simulink model "ramadan_2022"  (R2021a)
settings: Solver=ode15s  StartTime=0.0  StopTime=10  MaxStep=1e-2  MinStep=1e-20  RelTol=1e-3
StartFcn:
  | tic
StopFcn:
  | toc
  | 
  | 
  | %if GimbalLockFlag
  |  % fprintf(2, 'Almost reached Gimbal Lock of IMU. Simulation stopped.\n')
  | %end
  | 
  | %fprintf('Elapsed time: %4.2f sec (%4.2f%% realtime)\n', a, tout(end)/a*100)
values from neighbouring files (symbols this model uses):
  Balance = pMod(26:29)    [AssignSimulinkParams.m]    (also in assign_parameters.m = param(26:29))
  BalanceTrunkLat = pMod(22:25)    [AssignSimulinkParams.m]    (also in assign_parameters.m = param(22:25))
  BasisStim = pMod(1:11)    [AssignSimulinkParams.m]    (also in assign_parameters.m = param(1:11))
  CompliantLeg = pMod(12:14)    [AssignSimulinkParams.m]    (also in assign_parameters.m = param(12:14))
  CompliantLegLat = pMod(15)    [AssignSimulinkParams.m]    (also in assign_parameters.m = param(15))
  lp1 = 0.45    [nms3D_prep.m]
  lp2 = 0.55    [nms3D_prep.m]
  N = size(x,1)    [cmaes_hg.m]
  PreventKneeOverextension = pMod(16:21)    [AssignSimulinkParams.m]    (also in assign_parameters.m = param(16:21))
  propulsion = pMod(35)    [AssignSimulinkParams.m]    (also in assign_parameters.m = param(35))
  s = x(1:N-1,:).^2 + x(2:N,:).^2    [cmaes_hg.m]
  Target02 = pMod(30)    [AssignSimulinkParams.m]    (also in assign_parameters.m = param(30))
  Target13 = pMod(31:33)    [AssignSimulinkParams.m]    (also in assign_parameters.m = param(31:33))
  theta0 = pMod(34)    [AssignSimulinkParams.m]    (also in assign_parameters.m = param(34))
  WramameiSL_1000 = readmatrix('WSL_1000_Norm_Sigmoid_MSE_cont.csv')    [nms3D_prep.m]
  ZramameiSL_1000 = readmatrix('ZSL_1000_Norm_Sigmoid_MSE_cont.csv')    [nms3D_prep.m]
undefined symbols (not defined in the file or in its folder): ICs, mParams, X, Y, Z
libraries: nesl_utility x110, sm_lib x88, simulink x79, eeGeneralControl x28, robotmaniplib x10, dspinverses x10, robotcorelib x5, dspmathops x3, pid_lib x2, vrlib x1
(part 6 of 9)

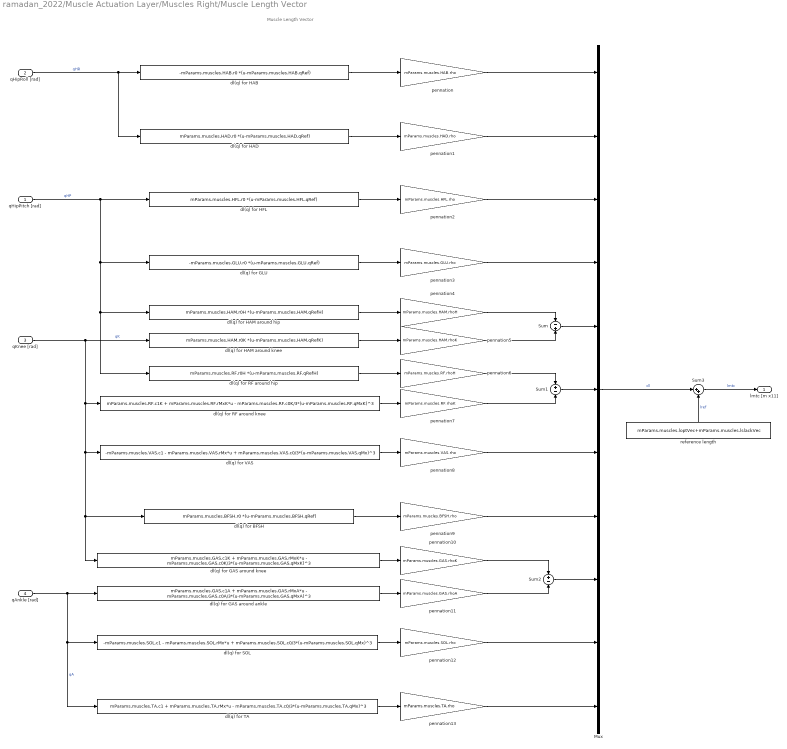
== system ramadan_2022/Muscle Actuation Layer/Muscles Right/Muscle Length Vector ==
  note: Muscle Length Vector
  qHipPitch [rad] : Inport
  qHipRoll [rad] : Inport  Port=2
  qKnee [rad] : Inport  Port=3
  qAnkle [rad] : Inport  Port=4
  Mux : Mux  Inputs=11
  Sum : Sum  Inputs=-+
  Sum1 : Sum  Inputs=+-
  Sum2 : Sum  Inputs=+-
  Sum3 : Sum  Inputs=|++
  dl(q) for BFSH : Fcn  Expr=mParams.muscles.BFSH.r0 *(u-mParams.muscles.BFSH.qRef)
  dl(q) for GAS around ankle : Fcn  Expr=mParams.muscles.GAS.c1A + mParams.muscles.GAS.rMxA*u - mParams.muscles.GAS.c0A/3*(u-mParams.muscles.GAS.qMxA)^3
  dl(q) for GAS around knee : Fcn  Expr=mParams.muscles.GAS.c1K + mParams.muscles.GAS.rMxK*u - mParams.muscles.GAS.c0K/3*(u-mParams.muscles.GAS.qMxK)^3
  dl(q) for GLU : Fcn  Expr=-mParams.muscles.GLU.r0 *(u-mParams.muscles.GLU.qRef)
  dl(q) for HAB : Fcn  Expr=-mParams.muscles.HAB.r0 *(u-mParams.muscles.HAB.qRef)
  dl(q) for HAD : Fcn  Expr=mParams.muscles.HAD.r0 *(u-mParams.muscles.HAD.qRef)
  dl(q) for HAM around hip : Fcn  Expr=mParams.muscles.HAM.r0H *(u-mParams.muscles.HAM.qRefH)
  dl(q) for HAM around knee : Fcn  Expr=mParams.muscles.HAM.r0K *(u-mParams.muscles.HAM.qRefK)
  dl(q) for HFL : Fcn  Expr=mParams.muscles.HFL.r0 *(u-mParams.muscles.HFL.qRef)
  dl(q) for RF around hip : Fcn  Expr=mParams.muscles.RF.r0H *(u-mParams.muscles.RF.qRefH)
  dl(q) for RF around knee : Fcn  Expr=mParams.muscles.RF.c1K + mParams.muscles.RF.rMxK*u - mParams.muscles.RF.c0K/3*(u-mParams.muscles.RF.qMxK)^3
  dl(q) for SOL : Fcn  Expr=-mParams.muscles.SOL.c1 - mParams.muscles.SOL.rMx*u + mParams.muscles.SOL.c0/3*(u-mParams.muscles.SOL.qMx)^3
  dl(q) for TA : Fcn  Expr=mParams.muscles.TA.c1 + mParams.muscles.TA.rMx*u - mParams.muscles.TA.c0/3*(u-mParams.muscles.TA.qMx)^3
  dl(q) for VAS : Fcn  Expr=-mParams.muscles.VAS.c1 - mParams.muscles.VAS.rMx*u + mParams.muscles.VAS.c0/3*(u-mParams.muscles.VAS.qMx)^3
  pennation : Gain  Gain=mParams.muscles.HAB.rho
  pennation1 : Gain  Gain=mParams.muscles.HAD.rho
  pennation10 : Gain  Gain=mParams.muscles.GAS.rhoK
  pennation11 : Gain  Gain=mParams.muscles.GAS.rhoA
  pennation12 : Gain  Gain=mParams.muscles.SOL.rho
  pennation13 : Gain  Gain=mParams.muscles.TA.rho
  pennation2 : Gain  Gain=mParams.muscles.HFL.rho
  pennation3 : Gain  Gain=mParams.muscles.GLU.rho
  pennation4 : Gain  Gain=mParams.muscles.HAM.rhoH
  pennation5 : Gain  Gain=mParams.muscles.HAM.rhoK
  pennation6 : Gain  Gain=mParams.muscles.RF.rhoH
  pennation7 : Gain  Gain=mParams.muscles.RF.rhoK
  pennation8 : Gain  Gain=mParams.muscles.VAS.rho
  pennation9 : Gain  Gain=mParams.muscles.BFSH.rho
  reference length : Constant  Value=mParams.muscles.loptVec+mParams.muscles.lslackVec
  lmtc [m x11] : Outport  VectorParamsAs1DForOutWhenUnconnected=off
  wires:
  dl(q) for HAB/1 -> pennation/1
  dl(q) for HFL/1 -> pennation2/1
  dl(q) for HAM around knee/1 -> pennation5/1
  dl(q) for BFSH/1 -> pennation9/1
  dl(q) for HAM around hip/1 -> pennation4/1
  qAnkle [rad]/1 -> dl(q) for TA/1, dl(q) for SOL/1, dl(q) for GAS around ankle/1  "qA"
  dl(q) for TA/1 -> pennation13/1
  dl(q) for HAD/1 -> pennation1/1
  dl(q) for GLU/1 -> pennation3/1
  dl(q) for RF around knee/1 -> pennation7/1
  dl(q) for SOL/1 -> pennation12/1
  qHipPitch [rad]/1 -> dl(q) for HAM around hip/1, dl(q) for RF around hip/1, dl(q) for GLU/1, dl(q) for HFL/1  "qHP"
  dl(q) for RF around hip/1 -> pennation6/1
  qHipRoll [rad]/1 -> dl(q) for HAD/1, dl(q) for HAB/1  "qHR"
  Sum1/1 -> Mux/6
  qKnee [rad]/1 -> dl(q) for HAM around knee/1, dl(q) for VAS/1, dl(q) for GAS around knee/1, dl(q) for BFSH/1, dl(q) for RF around knee/1  "qK"
  Sum/1 -> Mux/5
  Sum2/1 -> Mux/9
  dl(q) for GAS around knee/1 -> pennation10/1
  dl(q) for GAS around ankle/1 -> pennation11/1
  dl(q) for VAS/1 -> pennation8/1
  Mux/1 -> Sum3/1  "dl"
  Sum3/1 -> lmtc [m x11]/1  "lmtc"
  reference length/1 -> Sum3/2  "lref"
  pennation2/1 -> Mux/3
  pennation3/1 -> Mux/4
  pennation4/1 -> Sum/1
  pennation5/1 -> Sum/2
  pennation6/1 -> Sum1/1
  pennation7/1 -> Sum1/2
  pennation8/1 -> Mux/7
  pennation9/1 -> Mux/8
  pennation10/1 -> Sum2/1
  pennation11/1 -> Sum2/2
  pennation12/1 -> Mux/10
  pennation13/1 -> Mux/11
  pennation/1 -> Mux/1
  pennation1/1 -> Mux/2

== system ramadan_2022/Muscle Actuation Layer/Muscles Right/Muscle Torque Contributions ==
  note: Leg Muscle Torque Contributions
  qKnee [rad] : Inport
  qAnkle [rad] : Inport  Port=2
  FmVec [N x11] : Inport  Port=3
  Demux1 : Demux  Outputs=11
  Product{1..6} (6 alike) : Product
  Subsystem : Subsystem
  Sum : Sum  Inputs=+-
  Sum1 : Sum  Inputs=-++-
  Sum2 : Sum  Inputs=-++--
  Sum3 : Sum  Inputs=++-
  r(q) RF around knee : Fcn  Expr=mParams.muscles.RF.rMxK - mParams.muscles.RF.c0K*(u-mParams.muscles.RF.qMxK)^2
  r(q) RGAS around ankle : Fcn  Expr=mParams.muscles.GAS.rMxA - mParams.muscles.GAS.c0A*(u-mParams.muscles.GAS.qMxA)^2
  r(q) RGAS around knee : Fcn  Expr=mParams.muscles.GAS.rMxK - mParams.muscles.GAS.c0K*(u-mParams.muscles.GAS.qMxK)^2
  r(q) RSOL : Fcn  Expr=mParams.muscles.SOL.rMx - mParams.muscles.SOL.c0*(u-mParams.muscles.SOL.qMx)^2
  r(q) RTA : Fcn  Expr=mParams.muscles.TA.rMx - mParams.muscles.TA.c0*(u-mParams.muscles.TA.qMx)^2
  r(q) for BFSH : Gain  Gain=mParams.muscles.BFSH.r0
  r(q) for GLU : Gain  Gain=mParams.muscles.GLU.r0
  r(q) for HAB : Gain  Gain=mParams.muscles.HAB.r0
  r(q) for HAD : Gain  Gain=mParams.muscles.HAD.r0
  r(q) for HAM at hip : Gain  Gain=mParams.muscles.HAM.r0H
  r(q) for HAM at knee : Gain  Gain=mParams.muscles.HAM.r0K
  r(q) for HFL : Gain  Gain=mParams.muscles.HFL.r0
  r(q) for RF : Gain  Gain=mParams.muscles.RF.r0H
  r(q) for VAS : Fcn  Expr=mParams.muscles.VAS.rMx - mParams.muscles.VAS.c0*(u-mParams.muscles.VAS.qMx)^2
  tauHP [Nm] : Outport  VectorParamsAs1DForOutWhenUnconnected=off
  tauHR [Nm] : Outport  Port=2  VectorParamsAs1DForOutWhenUnconnected=off
  tauK [Nm] : Outport  Port=3  VectorParamsAs1DForOutWhenUnconnected=off
  tauA [Nm] : Outport  Port=4  VectorParamsAs1DForOutWhenUnconnected=off
  Leg Torque : Outport  Port=5  VectorParamsAs1DForOutWhenUnconnected=off
  wires:
  qKnee [rad]/1 -> r(q) RGAS around knee/1, r(q) RF around knee/1, r(q) for VAS/1  "qK"
  qAnkle [rad]/1 -> r(q) RTA/1, r(q) RSOL/1, r(q) RGAS around ankle/1  "qA"
  FmVec [N x11]/1 -> Demux1/1
  Demux1/1 -> r(q) for HAB/1  "HAB"
  Demux1/2 -> r(q) for HAD/1  "HAD"
  r(q) for HAD/1 -> Sum/2
  r(q) for HAB/1 -> Sum/1
  Demux1/3 -> r(q) for HFL/1  "HFL"
  Demux1/4 -> r(q) for GLU/1  "GLU"
  Demux1/5 -> r(q) for HAM at knee/1, r(q) for HAM at hip/1  "HAM"
  Demux1/6 -> Product1/1, r(q) for RF/1  "RF"
  r(q) for RF/1 -> Sum1/4
  r(q) RF around knee/1 -> Product1/2
  Product1/1 -> Sum2/2
  r(q) for HAM at knee/1 -> Sum2/1
  r(q) for HAM at hip/1 -> Sum1/3
  r(q) for GLU/1 -> Sum1/2
  r(q) for HFL/1 -> Sum1/1
  Sum1/1 -> tauHP [Nm]/1
  Demux1/7 -> Subsystem/1(F VAS), Product2/1  "VAS"
  Demux1/8 -> r(q) for BFSH/1  "BFSH"
  Demux1/9 -> Product3/1, Product4/1  "GAS"
  r(q) RGAS around knee/1 -> Product3/2
  Product2/1 -> Sum2/3
  r(q) for BFSH/1 -> Sum2/4
  Product3/1 -> Sum2/5
  Sum2/1 -> tauK [Nm]/1
  r(q) RGAS around ankle/1 -> Product4/2
  Demux1/10 -> Subsystem/3(F SOL), Product5/1  "SOL"
  r(q) RTA/1 -> Product6/2
  Demux1/11 -> Product6/1  "TA"
  Sum3/1 -> tauA [Nm]/1
  Sum/1 -> tauHR [Nm]/1
  Product6/1 -> Sum3/3
  Product4/1 -> Sum3/1
  Product5/1 -> Sum3/2
  r(q) for VAS/1 -> Subsystem/2(Moment Arm VAS), Product2/2
  r(q) RSOL/1 -> Subsystem/4(Moment Arm SOL), Product5/2
  Subsystem/1("Leg Torque ") -> Leg Torque/1

== system ramadan_2022/Spinal Layer/Stance Leg Control Left/L Stance Phase (coronal) ==
  note: Left Stance Phase Control
  note: M3: balance trunk old
  CompliantLegLat : Inport
  FmHAB : Inport  Port=2
  theta_tgt [rad] world : Inport  Port=3
  theta dtheta [rad rad/s] : Inport  Port=4
  BalanceTrunkLat old : Inport  Port=5
  Enable : EnablePort  StatesWhenEnabling=reset  ZeroCross=off
  Demux1 : Demux
  Demux7 : Demux  Outputs=2
  Divide{1..2,6..7,15} (5 alike) : Product
  Gain1 : Gain  Gain=-1
  Gain3 : Gain  Gain=-1
  Gain4 : Gain
  Mux2 : Mux  Inputs=2
  Sum1 : Sum  Inputs=-+|  InputSameDT=on  SaturateOnIntegerOverflow=on  OutDataTypeStr=Inherit: Same as first input
  Sum5 : Sum  Inputs=|++  InputSameDT=on  SaturateOnIntegerOverflow=on  OutDataTypeStr=Inherit: Same as first input
  Sum6 : Sum  Inputs=|++  InputSameDT=on  SaturateOnIntegerOverflow=on  OutDataTypeStr=Inherit: Same as first input
  positive half3 : Saturate  UpperLimit=inf  LowerLimit=0  ZeroCross=off
  positive half4 : Saturate  UpperLimit=inf  LowerLimit=0  ZeroCross=off
  S_M1 [HAB] : Outport  OutputWhenDisabled=reset  InitialOutput=0  VectorParamsAs1DForOutWhenUnconnected=off
  S_M3 [HAB HAD] old : Outport  Port=2  OutputWhenDisabled=reset  InitialOutput=0  VectorParamsAs1DForOutWhenUnconnected=off
  wires:
  Divide7/1 -> S_M1 [HAB]/1  "HAB"
  FmHAB/1 -> Divide7/2
  CompliantLegLat/1 -> Divide7/1
  Gain1/1 -> Divide2/1
  theta dtheta [rad rad/s]/1 -> Demux7/1
  positive half4/1 -> Mux2/2
  positive half3/1 -> Mux2/1
  Sum5/1 -> positive half3/1  "HAB"
  Divide2/1 -> Sum5/1
  Gain3/1 -> Divide6/1
  Demux1/2 -> Divide6/2  "GainDTh_HAB"
  Demux1/4 -> Divide15/2  "GainDTh_HAD"
  Divide6/1 -> Sum5/2
  BalanceTrunkLat old/1 -> Demux1/1
  theta_tgt [rad] world/1 -> Sum1/1
  Divide1/1 -> Sum6/1
  Divide15/1 -> Sum6/2
  Demux7/1 -> Sum1/2  "theta"
  Demux1/1 -> Divide2/2  "GainTh_HAB"
  Sum1/1 -> Gain1/1, Divide1/1
  Mux2/1 -> Gain4/1
  Demux1/3 -> Divide1/2  "GainTh_HAD"
  Demux7/2 -> Gain3/1, Divide15/1  "dtheta"
  Sum6/1 -> positive half4/1  "HAD"
  Gain4/1 -> S_M3 [HAB HAD] old/1

== system ramadan_2022/Spinal Layer/Stance Leg Control Left/L Stance Phase (sagittal) ==
  note: M1: realize compliant leg
  note: M2: prevent knee overextension
  FmGLU : Inport
  FmHAM : Inport  Port=2
  FmVAS : Inport  Port=3
  LceBFSH : Inport  Port=4
  FmGAS : Inport  Port=5
  FmSOL : Inport  Port=6
  Compliant Leg : Inport  Port=7
  Prevent Knee Overextension : Inport  Port=8
  Enable : EnablePort  StatesWhenEnabling=reset  ZeroCross=off
  Demux3 : Demux  Outputs=3
  Demux8 : Demux  Outputs=6
  Divide{7..8,10..11,13..15} (7 alike) : Product
  Gain : Gain  Gain=-1
  Mux2 : Mux  Inputs=3
  Mux4 : Mux
  Sum3 : Sum  Inputs=-+|  InputSameDT=on  SaturateOnIntegerOverflow=on  OutDataTypeStr=Inherit: Same as first input
  Sum4 : Sum  Inputs=-+|  InputSameDT=on  SaturateOnIntegerOverflow=on  OutDataTypeStr=Inherit: Same as first input
  positive half3 : Saturate  UpperLimit=inf  LowerLimit=0  ZeroCross=off
  positive half4 : Saturate  UpperLimit=inf  LowerLimit=0  ZeroCross=off
  S_M1 [GLU VAS SOL] : Outport  OutputWhenDisabled=reset  InitialOutput=0  VectorParamsAs1DForOutWhenUnconnected=off
  S_M2 [HAM VAS BFSH GAS] : Outport  Port=2  OutputWhenDisabled=reset  InitialOutput=0  VectorParamsAs1DForOutWhenUnconnected=off
  wires:
  Demux3/2 -> Divide8/1  "FGain_VAS"
  Demux3/3 -> Divide10/1  "FGain_SOL"
  Divide10/1 -> Mux2/3  "SOL"
  Divide8/1 -> Mux2/2  "VAS"
  Demux3/1 -> Divide7/1  "FGain_GLU"
  Divide7/1 -> Mux2/1  "GLU"
  FmGLU/1 -> Divide7/2
  FmVAS/1 -> Divide8/2
  FmSOL/1 -> Divide10/2
  Prevent Knee Overextension/1 -> Demux8/1
  Sum3/1 -> positive half3/1
  Demux8/3 -> Divide15/2  "LGainBFSH_VAS"
  Demux8/5 -> Divide13/2  "LGain_BFSH"
  Demux8/6 -> Divide11/1  "FGain_GAS"
  positive half3/1 -> Divide15/1
  Demux8/2 -> Sum3/1  "loff_BFSH_VAS"
  Divide15/1 -> Gain/1
  Divide11/1 -> Mux4/4  "GAS"
  Demux8/1 -> Divide14/1  "FGain_HAM"
  Divide14/1 -> Mux4/1  "HAM"
  Gain/1 -> Mux4/2  "VAS"
  Sum4/1 -> positive half4/1
  positive half4/1 -> Divide13/1
  Demux8/4 -> Sum4/1  "loff_BFSH"
  FmHAM/1 -> Divide14/2
  LceBFSH/1 -> Sum3/2, Sum4/2
  FmGAS/1 -> Divide11/2
  Mux4/1 -> S_M2 [HAM VAS BFSH GAS]/1
  Compliant Leg/1 -> Demux3/1
  Mux2/1 -> S_M1 [GLU VAS SOL]/1
  Divide13/1 -> Mux4/3  "BFSH"

== system ramadan_2022/Spinal Layer/Stance Leg Control Right/R Stance Phase (coronal) ==
  note: Left Stance Phase Control
  note: M3: balance trunk old
  CompliantLegLat : Inport
  FmHAB : Inport  Port=2
  theta_tgt [rad] world : Inport  Port=3
  theta dtheta [rad rad/s] : Inport  Port=4
  BalanceTrunkLat old : Inport  Port=5
  Enable : EnablePort  StatesWhenEnabling=reset  ZeroCross=off
  Demux1 : Demux
  Demux7 : Demux  Outputs=2
  Divide{1..2,6..7,15} (5 alike) : Product
  Gain1 : Gain  Gain=-1
  Gain3 : Gain  Gain=-1
  Gain4 : Gain
  Mux2 : Mux  Inputs=2
  Sum1 : Sum  Inputs=-+|  InputSameDT=on  SaturateOnIntegerOverflow=on  OutDataTypeStr=Inherit: Same as first input
  Sum5 : Sum  Inputs=|++  InputSameDT=on  SaturateOnIntegerOverflow=on  OutDataTypeStr=Inherit: Same as first input
  Sum6 : Sum  Inputs=|++  InputSameDT=on  SaturateOnIntegerOverflow=on  OutDataTypeStr=Inherit: Same as first input
  positive half3 : Saturate  UpperLimit=inf  LowerLimit=0  ZeroCross=off
  positive half4 : Saturate  UpperLimit=inf  LowerLimit=0  ZeroCross=off
  S_M1 [HAB] : Outport  OutputWhenDisabled=reset  InitialOutput=0  VectorParamsAs1DForOutWhenUnconnected=off
  S_M3 [HAB HAD] old : Outport  Port=2  OutputWhenDisabled=reset  InitialOutput=0  VectorParamsAs1DForOutWhenUnconnected=off
  wires:
  Divide7/1 -> S_M1 [HAB]/1  "HAB"
  FmHAB/1 -> Divide7/2
  CompliantLegLat/1 -> Divide7/1
  Gain1/1 -> Divide2/1
  theta dtheta [rad rad/s]/1 -> Demux7/1
  positive half4/1 -> Mux2/2
  positive half3/1 -> Mux2/1
  Sum5/1 -> positive half3/1  "HAB"
  Divide2/1 -> Sum5/1
  Gain3/1 -> Divide6/1
  Demux1/2 -> Divide6/2  "GainDTh_HAB"
  Demux1/4 -> Divide15/2  "GainDTh_HAD"
  Divide6/1 -> Sum5/2
  BalanceTrunkLat old/1 -> Demux1/1
  theta_tgt [rad] world/1 -> Sum1/1
  Divide1/1 -> Sum6/1
  Divide15/1 -> Sum6/2
  Demux7/1 -> Sum1/2  "theta"
  Demux1/1 -> Divide2/2  "GainTh_HAB"
  Sum1/1 -> Gain1/1, Divide1/1
  Mux2/1 -> Gain4/1
  Demux1/3 -> Divide1/2  "GainTh_HAD"
  Demux7/2 -> Gain3/1, Divide15/1  "dtheta"
  Sum6/1 -> positive half4/1  "HAD"
  Gain4/1 -> S_M3 [HAB HAD] old/1

== system ramadan_2022/Spinal Layer/Stance Leg Control Right/R Stance Phase (sagittal) ==
  note: M1: realize compliant leg
  note: M2: prevent knee overextension
  FmGLU : Inport
  FmHAM : Inport  Port=2
  FmVAS : Inport  Port=3
  LceBFSH : Inport  Port=4
  FmGAS : Inport  Port=5
  FmSOL : Inport  Port=6
  Compliant Leg : Inport  Port=7
  Prevent Knee Overextension : Inport  Port=8
  Enable : EnablePort  StatesWhenEnabling=reset  ZeroCross=off
  Demux3 : Demux  Outputs=3
  Demux8 : Demux  Outputs=6
  Divide{7..8,10..11,13..15} (7 alike) : Product
  Gain : Gain  Gain=-1
  Mux2 : Mux  Inputs=3
  Mux4 : Mux
  Sum3 : Sum  Inputs=-+|  InputSameDT=on  SaturateOnIntegerOverflow=on  OutDataTypeStr=Inherit: Same as first input
  Sum4 : Sum  Inputs=-+|  InputSameDT=on  SaturateOnIntegerOverflow=on  OutDataTypeStr=Inherit: Same as first input
  positive half3 : Saturate  UpperLimit=inf  LowerLimit=0  ZeroCross=off
  positive half4 : Saturate  UpperLimit=inf  LowerLimit=0  ZeroCross=off
  S_M1 [GLU VAS SOL] : Outport  OutputWhenDisabled=reset  InitialOutput=0  VectorParamsAs1DForOutWhenUnconnected=off
  S_M2 [HAM VAS BFSH GAS] : Outport  Port=2  OutputWhenDisabled=reset  InitialOutput=0  VectorParamsAs1DForOutWhenUnconnected=off
  wires:
  Demux3/2 -> Divide8/1  "FGain_VAS"
  Demux3/3 -> Divide10/1  "FGain_SOL"
  Divide10/1 -> Mux2/3  "SOL"
  Divide8/1 -> Mux2/2  "VAS"
  Demux3/1 -> Divide7/1  "FGain_GLU"
  Divide7/1 -> Mux2/1  "GLU"
  FmGLU/1 -> Divide7/2
  FmVAS/1 -> Divide8/2
  FmSOL/1 -> Divide10/2
  Prevent Knee Overextension/1 -> Demux8/1
  Sum3/1 -> positive half3/1
  Demux8/3 -> Divide15/2  "LGainBFSH_VAS"
  Demux8/5 -> Divide13/2  "LGain_BFSH"
  Demux8/6 -> Divide11/1  "FGain_GAS"
  positive half3/1 -> Divide15/1
  Demux8/2 -> Sum3/1  "loff_BFSH_VAS"
  Divide15/1 -> Gain/1
  Divide11/1 -> Mux4/4  "GAS"
  Demux8/1 -> Divide14/1  "FGain_HAM"
  Divide14/1 -> Mux4/1  "HAM"
  Gain/1 -> Mux4/2  "VAS"
  Sum4/1 -> positive half4/1
  positive half4/1 -> Divide13/1
  Demux8/4 -> Sum4/1  "loff_BFSH"
  FmHAM/1 -> Divide14/2
  LceBFSH/1 -> Sum3/2, Sum4/2
  FmGAS/1 -> Divide11/2
  Mux4/1 -> S_M2 [HAM VAS BFSH GAS]/1
  Compliant Leg/1 -> Demux3/1
  Mux2/1 -> S_M1 [GLU VAS SOL]/1
  Divide13/1 -> Mux4/3  "BFSH"

== system ramadan_2022/Spinal Layer/Stretch Reflex for Swing Leg Control/Stretch Reflex Left ==
  lambda : Inport
  l_ce : Inport  Port=2
  v_ce : Inport  Port=3
  lambda_dot : Inport  Port=4
  Add2 : Sum  Inputs=-+
  Add3 : Sum  Inputs=-+
  Add7 : Sum
  Gain10 : Gain  Gain=0.03
  Gain9 : Gain  Gain=mParams.muscles.K
  STIM : Outport  VectorParamsAs1DForOutWhenUnconnected=off
  wires:
  lambda/1 -> Add2/1
  Add7/1 -> STIM/1
  Gain9/1 -> Add7/1
  Gain10/1 -> Add7/2
  Add3/1 -> Gain10/1
  Add2/1 -> Gain9/1
  v_ce/1 -> Add3/2
  l_ce/1 -> Add2/2
  lambda_dot/1 -> Add3/1

== system ramadan_2022/Spinal Layer/Stretch Reflex for Swing Leg Control/Stretch Reflex Right ==
  lambda : Inport
  l_ce : Inport  Port=2
  v_ce : Inport  Port=3
  lambda_dot : Inport  Port=4
  Add2 : Sum  Inputs=-+
  Add3 : Sum  Inputs=-+
  Add7 : Sum
  Gain1 : Gain  Commented=on  Gain=[ 0.03 0.03 0.03 0.03 0.03 0.03 0.03 0.03 0.1 0.1 0.1]
  Gain10 : Gain  Gain=0.03
  Gain9 : Gain  Gain=mParams.muscles.K
  STIM : Outport  VectorParamsAs1DForOutWhenUnconnected=off
  wires:
  lambda/1 -> Add2/1
  Add7/1 -> STIM/1
  Gain9/1 -> Add7/1
  Gain10/1 -> Add7/2
  Add3/1 -> Gain10/1
  Add2/1 -> Gain9/1
  v_ce/1 -> Add3/2
  l_ce/1 -> Add2/2
  lambda_dot/1 -> Add3/1

== system ramadan_2022/Supraspinal Level/Subsystem/Compute positives forces that generate desired torque profiles ==
  note: Desired Forces: Desired Forces are computed by an iterative approach. The pseudoinverse-method is used to compute forces that generate the desired force profiles. This forces, however, can potentially be negative unlike real muscle forces. Therefore, torques that these negative forces would produce are computed. The resulting torques are again transformed into forces that have a smaller negative component now. This procedure is repeated 6 times.
  Left/Right : Inport
  Stance Left : Inport  Port=2
  Swing Left : Inport  Port=3
  Swing Right : Inport  Port=4
  Stance Right : Inport  Port=5
  Left : Subsystem
  Mux1 : Mux  Inputs=2
  Right : Subsystem
  Switch6 : Switch  Criteria=u2 > Threshold
  Switch7 : Switch  Criteria=u2 > Threshold
  Desired Force : Outport
  wires:
  ? -> ?
  [Llegq] -> Left/2(Angles)
  [Rlegq] -> Right/2(Angles)
  Switch6/1 -> Left/1(Desired Torques)
  Switch7/1 -> Right/1(Desired Torques)
  Swing Right/1 -> Switch7/1
  Swing Left/1 -> Switch6/3
  Stance Left/1 -> Switch6/1
  Stance Right/1 -> Switch7/3
  Left/1(Forces) -> Mux1/1
  Right/1(Forces) -> Mux1/2
  Mux1/1 -> Desired Force/1
  Left/Right/1 -> Switch6/2, Switch7/2

== system ramadan_2022/Supraspinal Level/Subsystem/Inversion of Muscle Model ==
  note: Inversion of Muscle Model: This block implements the inversion of the Hill-type muscle model.
  Desired Forces : Inport
  Demux : Demux  Outputs=22
  Divide1 : Product  Inputs=*/
  Divide11 : Product  Inputs=*/
  Fmax1 : Gain  Gain=1./mParams.muscles.FmaxVec  SaturateOnIntegerOverflow=on  OutDataTypeStr=Inherit: Same as input  ParamDataTypeStr=Inherit: Same as input
  Fmax4 : Gain  Gain=1./mParams.muscles.FmaxVec  SaturateOnIntegerOverflow=on  OutDataTypeStr=Inherit: Same as input  ParamDataTypeStr=Inherit: Same as input
  Multiply2 : Product
  Multiply6 : Product
  Mux : Mux  Inputs=11
  Mux1 : Mux  Inputs=11
  Saturation{1..3,5} (4 alike) : Saturate  UpperLimit=inf  LowerLimit=0.00005  ZeroCross=off
  Desired Activation Left : Outport
  Desired Activation Right : Outport  Port=2
  wires:
  Saturation1/1 -> Multiply6/1
  Demux/3 -> Mux/3
  Demux/9 -> Mux/9
  Demux/21 -> Mux1/10
  Demux/6 -> Mux/6
  Multiply6/1 -> Divide11/2
  Demux/11 -> Mux/11
  Demux/2 -> Mux/2
  Demux/7 -> Mux/7
  Mux/1 -> Fmax1/1
  Demux/19 -> Mux1/8
  Mux1/1 -> Fmax4/1
  [fl_R] -> Saturation2/1
  Desired Forces/1 -> Demux/1
  Demux/20 -> Mux1/9
  Demux/4 -> Mux/4
  [fl_L] -> Saturation5/1
  Demux/8 -> Mux/8
  Demux/1 -> Mux/1
  Demux/14 -> Mux1/3
  Demux/12 -> Mux1/1
  Fmax4/1 -> Divide11/1
  Saturation3/1 -> Multiply2/1
  [fv_R] -> Saturation1/1
  Demux/5 -> Mux/5
  Saturation5/1 -> Multiply2/2
  Demux/15 -> Mux1/4
  [fv_L] -> Saturation3/1
  Demux/18 -> Mux1/7
  Multiply2/1 -> Divide1/2
  Saturation2/1 -> Multiply6/2
  Demux/10 -> Mux/10
  Demux/16 -> Mux1/5
  Demux/22 -> Mux1/11
  Fmax1/1 -> Divide1/1
  Demux/13 -> Mux1/2
  Demux/17 -> Mux1/6
  Divide1/1 -> Desired Activation Left/1
  Divide11/1 -> Desired Activation Right/1

== system ramadan_2022/Supraspinal Level/Subsystem/Stance Leg2 ==
  note: Wrench to be generated by Left/Right Stance Leg
  Left/Right : Inport
  Balance Control Equation [Ankle Strategy] : Subsystem
  PD-Controller For Saggital Trunk Balance : Subsystem
  Stance Leg : Subsystem
  Push Off Left : Outport
  Push Off Right : Outport  Port=2
  wires:
  Left/Right/1 -> Stance Leg/1(left/right)
  Stance Leg/1(Push Off Left) -> Push Off Left/1
  Stance Leg/2(Push-Off Right) -> Push Off Right/1
  Balance Control Equation [Ankle Strategy]/1(Desired Acceleration (CoM)) -> Stance Leg/2(Balance Control [Ankle Strategy])
  PD-Controller For Saggital Trunk Balance/1(PD Input) -> Stance Leg/3(PD Input)

== system ramadan_2022/Supraspinal Level/Subsystem/Stretch Reflex Inversion ==
  note: Inversion of Stretch: This block implements the inversion of the tonic stretch reflex.
  Desired Activation Left : Inport
  Desired Activation Right : Inport  Port=2
  Gain1 : Gain  Gain=-1/mParams.muscles.K
  Gain12 : Gain  Gain=-1/mParams.muscles.K
  Sum14 : Sum  Inputs=|++
  Sum2 : Sum  Inputs=|++
  Descending Command Left : Outport
  Descending Command Right : Outport  Port=2
  wires:
  Desired Activation Right/1 -> Gain12/1
  Sum14/1 -> Descending Command Right/1
  Desired Activation Left/1 -> Gain1/1
  Sum2/1 -> Descending Command Left/1
  [RLceVec] -> Sum14/2
  Gain12/1 -> Sum14/1
  Gain1/1 -> Sum2/1
  [LLceVec] -> Sum2/2

== system ramadan_2022/Supraspinal Level/Subsystem/Swing Leg ==
  note: Target Joint Angles
  note: Movement Plan
  Left/Right : Inport
  Landing Preparation : Inport  Port=2
  Early/Late Swing : Inport  Port=3
  Check Quality Minimal Jerk : Subsystem
  Compute Acceleration Profiles with Minimal Jerk Approach : Subsystem
  Compute Acceleration Profiles with Minimal Jerk Approach1 : Subsystem  Commented=on
  Compute Target States : Subsystem
  Inverse Dynamics: Left Leg : Subsystem
  Inverse Dynamics: Right Leg : Subsystem
  Mux : Mux
  NOT : Logic  Operator=NOT  AllPortsSameDT=off  OutDataTypeStr=boolean
  NOT1 : Logic  Operator=NOT  AllPortsSameDT=off  OutDataTypeStr=boolean
  Product : Product
  Product1 : Product
  Scope2 : Scope
  Scope3 : Scope
  Scope4 : Scope
  Terminator : Terminator
  To Workspace2 : ToWorkspace  VariableName=Acceleration  SampleTime=-1
      settings: Save2DSignal=2-D array (concatenate along first dimension)
  To Workspace3 : ToWorkspace  VariableName=TargetStates  SampleTime=-1
      settings: Save2DSignal=2-D array (concatenate along first dimension)
  Desired Torques Left Swing : Outport
  Desired Torques Right Swing : Outport  Port=2
  Interaction Torques Left : Outport  Port=3
  Interaction Torques Right : Outport  Port=4
  wires:
  Inverse Dynamics: Left Leg/2(Interaction Wrench) -> Interaction Torques Left/1
  Inverse Dynamics: Right Leg/2(Interaction Wrench) -> Interaction Torques Right/1
  NOT/1 -> Inverse Dynamics: Left Leg/2(Enable)
  Inverse Dynamics: Right Leg/1(Desired Torques) -> Product/2, Scope4/1
  Mux/1 -> To Workspace3/1
  Early/Late Swing/1 -> Compute Target States/2(early/late), Compute Acceleration Profiles with Minimal Jerk Approach/6(Early/Late Swing)
  Compute Acceleration Profiles with Minimal Jerk Approach/1("Desired Acceleration ") -> To Workspace2/1, Scope2/1, Inverse Dynamics: Right Leg/1(Desired Acceleration), Inverse Dynamics: Left Leg/1(Desired Acceleration)
  Compute Acceleration Profiles with Minimal Jerk Approach/2(Joint Angles Swing) -> Terminator/1
  Inverse Dynamics: Left Leg/1(Desired Torques) -> Product1/1, Scope3/1
  Left/Right/1 -> NOT/1, Inverse Dynamics: Right Leg/2(Enable), Compute Acceleration Profiles with Minimal Jerk Approach/5(Swing Right/Left), Compute Target States/1(Left/Right)
  Landing Preparation/1 -> NOT1/1, Compute Acceleration Profiles with Minimal Jerk Approach/7(Landing Preparation)
  Compute Target States/4(Hip Roll Target) -> Mux/4, Check Quality Minimal Jerk/4(In4), Compute Acceleration Profiles with Minimal Jerk Approach/4(Target State Hip Roll)
  Compute Target States/1(Hip Pitch Target) -> Check Quality Minimal Jerk/1(In1), Compute Acceleration Profiles with Minimal Jerk Approach/1(Target State Hip Pitch), Mux/1
  Compute Target States/3(Ankle Target) -> Mux/3, Check Quality Minimal Jerk/3(In3), Compute Acceleration Profiles with Minimal Jerk Approach/3(Target State Ankle)
  Compute Target States/2(Knee Target) -> Mux/2, Check Quality Minimal Jerk/2(In2), Compute Acceleration Profiles with Minimal Jerk Approach/2(Target State Knee)
  Product/1 -> Desired Torques Right Swing/1
  Product1/1 -> Desired Torques Left Swing/1
  NOT1/1 -> Product/1, Product1/2

== system ramadan_2022/Body and Contact Model/L Leg/Foot/  XYZ Sensor Ball left1 ==
  note: Simplified IMU Model
  Frame Sensor : sm_lib/Frames and Transforms/Transform Sensor  MeasurementFrame=World  SenseAngle=off  SenseAxis=off  SenseAngle1=off  SenseAngle2=off  SenseAngle3=off  SenseQ=off  SenseR=on  SenseOmegaX=off  SenseOmegaY=off  SenseOmegaZ=off  SenseOmega1=off  SenseOmega2=off  SenseOmega3=off  SenseQDot=off  SenseRDot=off  SenseAlphaX=off  SenseAlphaY=off  SenseAlphaZ=off  SenseAlpha1=off  SenseAlpha2=off  SenseAlpha3=off  SenseQDDot=off  SenseRDDot=off  SenseX=on  SenseY=on  SenseZ=on  SenseRad=off  SenseAzim=off  SenseDist=off  SenseInc=off  SenseXDot=on  SenseYDot=on  SenseZDot=on  SenseRadDot=off  SenseAzimDot=off  SenseDistDot=off  SenseIncDot=off  SenseXDDot=off  SenseYDDot=off  SenseZDDot=off  SenseRadDDot=off  SenseAzimDDot=off  SenseDistDDot=off  SenseIncDDot=off
  Mux3 : Mux  Inputs=3
  Mux4 : Mux  Inputs=3
  PS-Simulink Converter : nesl_utility/PS-Simulink Converter  PhysicalDomain=network_engine_domain  SubClassName=ps_output  LeftPortType=input  RightPortType=output  PseudoPeriodic=off  Frequencies=[]  Unit=m  AffineConversion=off
      settings: SourceProductBaseCode=PW,SS
  PS-Simulink Converter1 : nesl_utility/PS-Simulink Converter  PhysicalDomain=network_engine_domain  SubClassName=ps_output  LeftPortType=input  RightPortType=output  PseudoPeriodic=off  Frequencies=[]  Unit=m  AffineConversion=off
      settings: SourceProductBaseCode=PW,SS
  PS-Simulink Converter2 : nesl_utility/PS-Simulink Converter  PhysicalDomain=network_engine_domain  SubClassName=ps_output  LeftPortType=input  RightPortType=output  PseudoPeriodic=off  Frequencies=[]  Unit=m/s  AffineConversion=off
      settings: SourceProductBaseCode=PW,SS
  PS-Simulink Converter3 : nesl_utility/PS-Simulink Converter  PhysicalDomain=network_engine_domain  SubClassName=ps_output  LeftPortType=input  RightPortType=output  PseudoPeriodic=off  Frequencies=[]  Unit=m/s  AffineConversion=off
      settings: SourceProductBaseCode=PW,SS
  PS-Simulink Converter4 : nesl_utility/PS-Simulink Converter  PhysicalDomain=network_engine_domain  SubClassName=ps_output  LeftPortType=input  RightPortType=output  PseudoPeriodic=off  Frequencies=[]  Unit=m  AffineConversion=off
      settings: SourceProductBaseCode=PW,SS
  PS-Simulink Converter5 : nesl_utility/PS-Simulink Converter  PhysicalDomain=network_engine_domain  SubClassName=ps_output  LeftPortType=input  RightPortType=output  PseudoPeriodic=off  Frequencies=[]  Unit=m/s  AffineConversion=off
      settings: SourceProductBaseCode=PW,SS
  PS-Simulink Converter6 : nesl_utility/PS-Simulink Converter  PhysicalDomain=network_engine_domain  SubClassName=ps_output  LeftPortType=input  RightPortType=output  PseudoPeriodic=off  Frequencies=[]  Unit=rad  AffineConversion=off
      settings: SourceProductBaseCode=PW,SS
  World Frame : sm_lib/Frames and Transforms/World Frame
  frame : PMIOPort  Side=Left
  p_bLH [m x3] : Outport  VectorParamsAs1DForOutWhenUnconnected=off
  v_bLH [m/s x3] : Outport  Port=2  VectorParamsAs1DForOutWhenUnconnected=off
  Rotation Matrix : Outport  Port=3  VectorParamsAs1DForOutWhenUnconnected=off
  wires:
  PS-Simulink Converter4/1 -> Mux3/3
  PS-Simulink Converter3/1 -> Mux4/2
  PS-Simulink Converter5/1 -> Mux4/3
  PS-Simulink Converter/1 -> Mux3/1
  Mux3/1 -> p_bLH [m x3]/1
  Mux4/1 -> v_bLH [m/s x3]/1
  PS-Simulink Converter2/1 -> Mux4/1
  PS-Simulink Converter1/1 -> Mux3/2
  PS-Simulink Converter6/1 -> Rotation Matrix/1
  connections:
  Frame Sensor/RConn1 -- frame/RConn1
  World Frame/RConn1 -- Frame Sensor/LConn1
  Frame Sensor/RConn3 -- PS-Simulink Converter/LConn1
  Frame Sensor/RConn4 -- PS-Simulink Converter1/LConn1
  Frame Sensor/RConn5 -- PS-Simulink Converter4/LConn1
  Frame Sensor/RConn6 -- PS-Simulink Converter2/LConn1
  Frame Sensor/RConn7 -- PS-Simulink Converter3/LConn1
  Frame Sensor/RConn8 -- PS-Simulink Converter5/LConn1
  Frame Sensor/RConn2 -- PS-Simulink Converter6/LConn1

== system ramadan_2022/Body and Contact Model/R Leg/Foot1/  XYZ Sensor  ==
  note: Simplified IMU Model
  Frame Sensor : sm_lib/Frames and Transforms/Transform Sensor  MeasurementFrame=World  SenseAngle=off  SenseAxis=off  SenseAngle1=off  SenseAngle2=off  SenseAngle3=off  SenseQ=off  SenseR=off  SenseOmegaX=off  SenseOmegaY=off  SenseOmegaZ=off  SenseOmega1=off  SenseOmega2=off  SenseOmega3=off  SenseQDot=off  SenseRDot=off  SenseAlphaX=off  SenseAlphaY=off  SenseAlphaZ=off  SenseAlpha1=off  SenseAlpha2=off  SenseAlpha3=off  SenseQDDot=off  SenseRDDot=off  SenseX=on  SenseY=on  SenseZ=on  SenseRad=off  SenseAzim=off  SenseDist=off  SenseInc=off  SenseXDot=on  SenseYDot=on  SenseZDot=on  SenseRadDot=off  SenseAzimDot=off  SenseDistDot=off  SenseIncDot=off  SenseXDDot=off  SenseYDDot=off  SenseZDDot=off  SenseRadDDot=off  SenseAzimDDot=off  SenseDistDDot=off  SenseIncDDot=off
  Mux3 : Mux  Inputs=3
  Mux4 : Mux  Inputs=3
  PS-Simulink Converter : nesl_utility/PS-Simulink Converter  PhysicalDomain=network_engine_domain  SubClassName=ps_output  LeftPortType=input  RightPortType=output  PseudoPeriodic=off  Frequencies=[]  Unit=m  AffineConversion=off
      settings: SourceProductBaseCode=PW,SS
  PS-Simulink Converter1 : nesl_utility/PS-Simulink Converter  PhysicalDomain=network_engine_domain  SubClassName=ps_output  LeftPortType=input  RightPortType=output  PseudoPeriodic=off  Frequencies=[]  Unit=m  AffineConversion=off
      settings: SourceProductBaseCode=PW,SS
  PS-Simulink Converter2 : nesl_utility/PS-Simulink Converter  PhysicalDomain=network_engine_domain  SubClassName=ps_output  LeftPortType=input  RightPortType=output  PseudoPeriodic=off  Frequencies=[]  Unit=m/s  AffineConversion=off
      settings: SourceProductBaseCode=PW,SS
  PS-Simulink Converter3 : nesl_utility/PS-Simulink Converter  PhysicalDomain=network_engine_domain  SubClassName=ps_output  LeftPortType=input  RightPortType=output  PseudoPeriodic=off  Frequencies=[]  Unit=m/s  AffineConversion=off
      settings: SourceProductBaseCode=PW,SS
  PS-Simulink Converter4 : nesl_utility/PS-Simulink Converter  PhysicalDomain=network_engine_domain  SubClassName=ps_output  LeftPortType=input  RightPortType=output  PseudoPeriodic=off  Frequencies=[]  Unit=m  AffineConversion=off
      settings: SourceProductBaseCode=PW,SS
  PS-Simulink Converter5 : nesl_utility/PS-Simulink Converter  PhysicalDomain=network_engine_domain  SubClassName=ps_output  LeftPortType=input  RightPortType=output  PseudoPeriodic=off  Frequencies=[]  Unit=m/s  AffineConversion=off
      settings: SourceProductBaseCode=PW,SS
  World Frame : sm_lib/Frames and Transforms/World Frame
  frame : PMIOPort  Side=Left
  p_bLH [m x3] : Outport  VectorParamsAs1DForOutWhenUnconnected=off
  v_bLH [m/s x3] : Outport  Port=2  VectorParamsAs1DForOutWhenUnconnected=off
  wires:
  PS-Simulink Converter4/1 -> Mux3/3
  PS-Simulink Converter3/1 -> Mux4/2
  PS-Simulink Converter5/1 -> Mux4/3
  PS-Simulink Converter/1 -> Mux3/1
  Mux3/1 -> p_bLH [m x3]/1
  Mux4/1 -> v_bLH [m/s x3]/1
  PS-Simulink Converter2/1 -> Mux4/1
  PS-Simulink Converter1/1 -> Mux3/2
  connections:
  Frame Sensor/RConn1 -- frame/RConn1
  World Frame/RConn1 -- Frame Sensor/LConn1
  Frame Sensor/RConn2 -- PS-Simulink Converter/LConn1
  Frame Sensor/RConn3 -- PS-Simulink Converter1/LConn1
  Frame Sensor/RConn4 -- PS-Simulink Converter4/LConn1
  Frame Sensor/RConn5 -- PS-Simulink Converter2/LConn1
  Frame Sensor/RConn6 -- PS-Simulink Converter3/LConn1
  Frame Sensor/RConn7 -- PS-Simulink Converter5/LConn1

== system ramadan_2022/Body and Contact Model/R Leg/Foot1/  XYZ Sensor Ball left1 ==
  note: Simplified IMU Model
  Frame Sensor : sm_lib/Frames and Transforms/Transform Sensor  MeasurementFrame=World  SenseAngle=off  SenseAxis=off  SenseAngle1=off  SenseAngle2=off  SenseAngle3=off  SenseQ=off  SenseR=on  SenseOmegaX=off  SenseOmegaY=off  SenseOmegaZ=off  SenseOmega1=off  SenseOmega2=off  SenseOmega3=off  SenseQDot=off  SenseRDot=off  SenseAlphaX=off  SenseAlphaY=off  SenseAlphaZ=off  SenseAlpha1=off  SenseAlpha2=off  SenseAlpha3=off  SenseQDDot=off  SenseRDDot=off  SenseX=on  SenseY=on  SenseZ=on  SenseRad=off  SenseAzim=off  SenseDist=off  SenseInc=off  SenseXDot=on  SenseYDot=on  SenseZDot=on  SenseRadDot=off  SenseAzimDot=off  SenseDistDot=off  SenseIncDot=off  SenseXDDot=off  SenseYDDot=off  SenseZDDot=off  SenseRadDDot=off  SenseAzimDDot=off  SenseDistDDot=off  SenseIncDDot=off
  Mux3 : Mux  Inputs=3
  Mux4 : Mux  Inputs=3
  PS-Simulink Converter : nesl_utility/PS-Simulink Converter  PhysicalDomain=network_engine_domain  SubClassName=ps_output  LeftPortType=input  RightPortType=output  PseudoPeriodic=off  Frequencies=[]  Unit=m  AffineConversion=off
      settings: SourceProductBaseCode=PW,SS
  PS-Simulink Converter1 : nesl_utility/PS-Simulink Converter  PhysicalDomain=network_engine_domain  SubClassName=ps_output  LeftPortType=input  RightPortType=output  PseudoPeriodic=off  Frequencies=[]  Unit=m  AffineConversion=off
      settings: SourceProductBaseCode=PW,SS
  PS-Simulink Converter2 : nesl_utility/PS-Simulink Converter  PhysicalDomain=network_engine_domain  SubClassName=ps_output  LeftPortType=input  RightPortType=output  PseudoPeriodic=off  Frequencies=[]  Unit=m/s  AffineConversion=off
      settings: SourceProductBaseCode=PW,SS
  PS-Simulink Converter3 : nesl_utility/PS-Simulink Converter  PhysicalDomain=network_engine_domain  SubClassName=ps_output  LeftPortType=input  RightPortType=output  PseudoPeriodic=off  Frequencies=[]  Unit=m/s  AffineConversion=off
      settings: SourceProductBaseCode=PW,SS
  PS-Simulink Converter4 : nesl_utility/PS-Simulink Converter  PhysicalDomain=network_engine_domain  SubClassName=ps_output  LeftPortType=input  RightPortType=output  PseudoPeriodic=off  Frequencies=[]  Unit=m  AffineConversion=off
      settings: SourceProductBaseCode=PW,SS
  PS-Simulink Converter5 : nesl_utility/PS-Simulink Converter  PhysicalDomain=network_engine_domain  SubClassName=ps_output  LeftPortType=input  RightPortType=output  PseudoPeriodic=off  Frequencies=[]  Unit=m/s  AffineConversion=off
      settings: SourceProductBaseCode=PW,SS
  PS-Simulink Converter6 : nesl_utility/PS-Simulink Converter  PhysicalDomain=network_engine_domain  SubClassName=ps_output  LeftPortType=input  RightPortType=output  PseudoPeriodic=off  Frequencies=[]  Unit=rad  AffineConversion=off
      settings: SourceProductBaseCode=PW,SS
  World Frame : sm_lib/Frames and Transforms/World Frame
  frame : PMIOPort  Side=Left
  p_bLH [m x3] : Outport  VectorParamsAs1DForOutWhenUnconnected=off
  v_bLH [m/s x3] : Outport  Port=2  VectorParamsAs1DForOutWhenUnconnected=off
  Rotation Matrix : Outport  Port=3  VectorParamsAs1DForOutWhenUnconnected=off
  wires:
  PS-Simulink Converter4/1 -> Mux3/3
  PS-Simulink Converter3/1 -> Mux4/2
  PS-Simulink Converter5/1 -> Mux4/3
  PS-Simulink Converter/1 -> Mux3/1
  Mux3/1 -> p_bLH [m x3]/1
  Mux4/1 -> v_bLH [m/s x3]/1
  PS-Simulink Converter2/1 -> Mux4/1
  PS-Simulink Converter1/1 -> Mux3/2
  PS-Simulink Converter6/1 -> Rotation Matrix/1
  connections:
  Frame Sensor/RConn1 -- frame/RConn1
  World Frame/RConn1 -- Frame Sensor/LConn1
  Frame Sensor/RConn3 -- PS-Simulink Converter/LConn1
  Frame Sensor/RConn4 -- PS-Simulink Converter1/LConn1
  Frame Sensor/RConn5 -- PS-Simulink Converter4/LConn1
  Frame Sensor/RConn6 -- PS-Simulink Converter2/LConn1
  Frame Sensor/RConn7 -- PS-Simulink Converter3/LConn1
  Frame Sensor/RConn8 -- PS-Simulink Converter5/LConn1
  Frame Sensor/RConn2 -- PS-Simulink Converter6/LConn1

== system ramadan_2022/Body and Contact Model/Vestibular System/Align Axis/Compute Lateral Rotation ==
  Hip Left : Inport
  Hip Right : Inport  Port=2
  Constant : Constant  Value=[0 0 1]
  Constant1 : Constant
  Constant2 : Constant  Value=-1
  Dot Product : DotProduct  InputSameDT=on  OutDataTypeStr=Inherit: Inherit via internal rule
  Minus : Sum  Inputs=+-
  Normalization : dspmathops/Normalization  NormType=2-norm  Bias=1e-10  NormOver=Each column  Dimension=1  roundingMode=Floor  overflowMode=off  accumDataTypeStr=Inherit: Same as product output  accumLastDataTypeStr=Inherit: Same as product output  outputDataTypeStr=Inherit: Same as product output  outputMin=[]  outputMax=[]  outputLastDataTypeStr=Inherit: Same as product output
  Product : Product
  Selector : Selector  InputPortWidth=3  IndexOptions=Index vector (dialog)  Indices=[2]  OutputSizes=1
  Switch : Switch  Criteria=u2 > Threshold  ZeroCross=off
  Trigonometric Function : Trigonometry  Operator=acos
  Lateral Rotation : Outport
  wires:
  Hip Right/1 -> Minus/1
  Selector/1 -> Switch/2
  Product/1 -> Lateral Rotation/1
  Constant2/1 -> Switch/1
  Constant/1 -> Dot Product/1
  Constant1/1 -> Switch/3
  Switch/1 -> Product/1
  Trigonometric Function/1 -> Product/2
  Minus/1 -> Normalization/1
  Normalization/1 -> Dot Product/2, Selector/1
  Dot Product/1 -> Trigonometric Function/1
  Hip Left/1 -> Minus/2

== system ramadan_2022/Body and Contact Model/Vestibular System/Align Axis/Compute Saggital Rotation ==
  Hip Position Left [m] : Inport
  Hip Position Right [m] : Inport  Port=2
  Trunk Position [m] : Inport  Port=3
  Constant : Constant  Value=[0 1 0]
  Constant1 : Constant
  Constant2 : Constant  Value=-1
  Dot Product : DotProduct  InputSameDT=on  OutDataTypeStr=Inherit: Inherit via internal rule
  Gain : Gain  Gain=[0.5 0.5 0]
  Gain1 : Gain  Gain=[1 1 0]
  Minus : Sum
  Minus1 : Sum  Inputs=+-
  Normalization : dspmathops/Normalization  NormType=2-norm  Bias=1e-10  NormOver=Each column  Dimension=1  roundingMode=Floor  overflowMode=off  accumDataTypeStr=Inherit: Same as product output  accumLastDataTypeStr=Inherit: Same as product output  outputDataTypeStr=Inherit: Same as product output  outputMin=[]  outputMax=[]  outputLastDataTypeStr=Inherit: Same as product output
  Product : Product
  Selector : Selector  InputPortWidth=3  IndexOptions=Index vector (dialog)  Indices=[1]  OutputSizes=1
  Switch : Switch  Criteria=u2 > Threshold
  Trigonometric Function : Trigonometry  Operator=acos
  Saggital Rotation : Outport
  wires:
  Hip Position Right [m]/1 -> Minus/1
  Trigonometric Function/1 -> Product/2
  Constant/1 -> Dot Product/1
  Dot Product/1 -> Trigonometric Function/1
  Hip Position Left [m]/1 -> Minus/2
  Minus/1 -> Gain/1
  Gain/1 -> Minus1/2
  Trunk Position [m]/1 -> Gain1/1
  Minus1/1 -> Normalization/1
  Selector/1 -> Switch/2
  Constant1/1 -> Switch/3
  Constant2/1 -> Switch/1
  Switch/1 -> Product/1
  Product/1 -> Saggital Rotation/1
  Gain1/1 -> Minus1/1
  Normalization/1 -> Selector/1, Dot Product/2

== system ramadan_2022/Muscle Actuation Layer/Muscles Left/Muscle Dynamics (Vectorized)1/BE force-length relation ==
  note: Buffer Elasticity BE
  lce [lopt] : Inport
  Constant1 : Constant  Value=1-mParams.muscles.w
  Math Function : Math  Operator=square  SignedPower=on  SaturateOnIntegerOverflow=on
  Sum4 : Sum  Inputs=|+-  InputSameDT=on  SaturateOnIntegerOverflow=on  OutDataTypeStr=Inherit: Same as first input
  buffer engaged? : simulink/Logic and Bit Operations/Compare To Zero  relop=<  OutDataTypeStr=boolean  ZeroCross=off
  force of buffer elasticity : Product  Inputs=**
  reference strain [lslack] : Constant  Value=mParams.muscles.w/2
  relative strain : Product  Inputs=*/
  fbe [Fmax] : Outport  VectorParamsAs1DForOutWhenUnconnected=off
  wires:
  force of buffer elasticity/1 -> fbe [Fmax]/1
  Math Function/1 -> force of buffer elasticity/2
  buffer engaged?/1 -> force of buffer elasticity/1
  Constant1/1 -> Sum4/2
  Sum4/1 -> relative strain/1, buffer engaged?/1
  reference strain [lslack]/1 -> relative strain/2
  relative strain/1 -> Math Function/1
  lce [lopt]/1 -> Sum4/1

== system ramadan_2022/Muscle Actuation Layer/Muscles Left/Muscle Dynamics (Vectorized)1/CE force-length relation ==
  note: CE Force-Length Relationship
  lce [lopt] : Inport
  Abs : Abs  ZeroCross=off
  Constant1 : Constant
  Constant2 : Constant  Value=3
  Gain : Gain  Gain=log(mParams.muscles.c)
  Math Function : Math  SignedPower=on  SaturateOnIntegerOverflow=on
  Math Function1 : Math  Operator=pow  SignedPower=on  SaturateOnIntegerOverflow=on
  Sum4 : Sum  Inputs=|+-  InputSameDT=on  SaturateOnIntegerOverflow=on  OutDataTypeStr=Inherit: Same as first input
  normalized position : Product  Inputs=*/
  relative width : Constant  Value=mParams.muscles.w
  fce [Fmax] : Outport  VectorParamsAs1DForOutWhenUnconnected=off
  wires:
  Math Function/1 -> fce [Fmax]/1
  Gain/1 -> Math Function/1
  Math Function1/1 -> Gain/1
  Constant2/1 -> Math Function1/2
  normalized position/1 -> Math Function1/1
  Abs/1 -> normalized position/1
  Sum4/1 -> Abs/1
  Constant1/1 -> Sum4/2
  relative width/1 -> normalized position/2
  lce [lopt]/1 -> Sum4/1

== system ramadan_2022/Muscle Actuation Layer/Muscles Left/Muscle Dynamics (Vectorized)1/CE inverse force-velocity relation ==
  note: CE Inverse Force-Velocity Relationship
  Fv[Fmax] : Inport
  1 : Product  Inputs=/*
  Constant{1,3..4,8} (4 alike) : Constant
  Constant2 : Constant  Value=mParams.muscles.N
  Curvature : Gain  Gain=mParams.muscles.K  SaturateOnIntegerOverflow=on  OutDataTypeStr=Inherit: Same as input  ParamDataTypeStr=Inherit: Same as input
  Curvature1 : Gain  Gain=7.56*mParams.muscles.K  SaturateOnIntegerOverflow=on  OutDataTypeStr=Inherit: Same as input  ParamDataTypeStr=Inherit: Same as input
  Logical Operator : Logic  Operator=NOT  AllPortsSameDT=off  OutDataTypeStr=boolean
  Logical Operator1 : Logic  Operator=NOT  AllPortsSameDT=off  OutDataTypeStr=boolean
  Slope : Gain  Gain=1e-2  SaturateOnIntegerOverflow=on  OutDataTypeStr=Inherit: Same as input  ParamDataTypeStr=Inherit: Same as input
  Sum1 : Sum  Inputs=|++  InputSameDT=on  SaturateOnIntegerOverflow=on  OutDataTypeStr=Inherit: Same as first input
  Sum2 : Sum  InputSameDT=on  SaturateOnIntegerOverflow=on  OutDataTypeStr=Inherit: Same as first input
  Sum3 : Sum  Inputs=++|  InputSameDT=on  SaturateOnIntegerOverflow=on  OutDataTypeStr=Inherit: Same as first input
  Sum4 : Sum  Inputs=|+-  InputSameDT=on  SaturateOnIntegerOverflow=on  OutDataTypeStr=Inherit: Same as first input
  Sum5 : Sum  Inputs=|-+  InputSameDT=on  SaturateOnIntegerOverflow=on  OutDataTypeStr=Inherit: Same as first input
  Sum6 : Sum  Inputs=-+|  InputSameDT=on  SaturateOnIntegerOverflow=on  OutDataTypeStr=Inherit: Same as first input
  Sum7 : Sum  Inputs=|++  InputSameDT=on  SaturateOnIntegerOverflow=on  OutDataTypeStr=Inherit: Same as first input
  Sum8 : Sum  Inputs=+-|  InputSameDT=on  SaturateOnIntegerOverflow=on  OutDataTypeStr=Inherit: Same as first input
  Sum9 : Sum  InputSameDT=on  SaturateOnIntegerOverflow=on  OutDataTypeStr=Inherit: Same as first input
  extension force within bound? : simulink/Logic and Bit Operations/Compare To Constant  relop=<=  const=mParams.muscles.N  OutDataTypeStr=boolean  ZeroCross=off
  force indicating contraction? : simulink/Logic and Bit Operations/Compare To Constant  relop=<=  const=1  OutDataTypeStr=boolean  ZeroCross=off
  v_concentric : Product  Inputs=*/
  v_concentric1 : Product  Inputs=**
  v_excentric <=N 1 : Product  Inputs=***
  v_excentric <N : Product  Inputs=*/
  v_excentric >N : Product  Inputs=**
  v[vmax] : Outport  VectorParamsAs1DForOutWhenUnconnected=off
  wires:
  Sum2/1 -> Sum9/2
  v_excentric <=N 1/1 -> Sum2/1
  Logical Operator1/1 -> v_excentric >N/1
  v_excentric >N/1 -> Sum2/2
  Logical Operator/1 -> v_excentric <=N 1/1
  Fv[Fmax]/1 -> extension force within bound?/1, force indicating contraction?/1, Curvature/1, Sum4/1, Sum6/2
  extension force within bound?/1 -> Logical Operator1/1, v_excentric <=N 1/3
  force indicating contraction?/1 -> Logical Operator/1, v_concentric1/2
  Sum1/1 -> v_excentric >N/2
  v_concentric1/1 -> Sum9/1
  v_excentric <N/1 -> v_excentric <=N 1/2
  Constant3/1 -> Sum5/1
  Sum5/1 -> 1/1
  Constant2/1 -> Sum5/2, Sum6/1
  Sum6/1 -> Slope/1, 1/2
  Constant8/1 -> Sum1/2
  Slope/1 -> Sum1/1
  Sum9/1 -> v[vmax]/1
  v_concentric/1 -> v_concentric1/1
  Sum7/1 -> v_excentric <N/1
  Sum8/1 -> v_excentric <N/2
  Curvature1/1 -> Sum8/2
  Constant4/1 -> Sum8/1, Sum7/2
  1/1 -> Curvature1/1, Sum7/1
  Sum3/1 -> v_concentric/2
  Sum4/1 -> v_concentric/1
  Constant1/1 -> Sum3/1, Sum4/2
  Curvature/1 -> Sum3/2

== system ramadan_2022/Muscle Actuation Layer/Muscles Left/Muscle Dynamics (Vectorized)1/PE force-length relation ==
  note: Parallel Elasticity PE
  lce [lopt] : Inport
  Constant3 : Constant
  Math Function2 : Math  Operator=square  SignedPower=on  SaturateOnIntegerOverflow=on
  Scope : Scope
  Scope1 : Scope
  Sum1 : Sum  Inputs=|+-  InputSameDT=on  SaturateOnIntegerOverflow=on  OutDataTypeStr=Inherit: Same as first input
  force of buffer elasticity : Product  Inputs=**
  parallel elasticity engaged? : simulink/Logic and Bit Operations/Compare To Zero  relop=>  OutDataTypeStr=boolean  ZeroCross=off
  reference strain [lopt] : Constant  Value=mParams.muscles.w
  relative strain : Product  Inputs=*/
  fpe [Fmax] : Outport  VectorParamsAs1DForOutWhenUnconnected=off
  wires:
  parallel elasticity engaged?/1 -> force of buffer elasticity/1
  force of buffer elasticity/1 -> fpe [Fmax]/1
  Math Function2/1 -> force of buffer elasticity/2
  relative strain/1 -> Math Function2/1
  reference strain [lopt]/1 -> relative strain/2
  Sum1/1 -> Scope/1, relative strain/1, parallel elasticity engaged?/1
  Constant3/1 -> Sum1/2
  lce [lopt]/1 -> Scope1/1, Sum1/1

== system ramadan_2022/Muscle Actuation Layer/Muscles Left/Muscle Dynamics (Vectorized)1/SE force-length relation ==
  note: SE Force-Length Relationship
  lse [lslack] : Inport
  Constant1 : Constant
  Math Function : Math  Operator=square  SignedPower=on  SaturateOnIntegerOverflow=on
  Sum4 : Sum  Inputs=|+-  InputSameDT=on  SaturateOnIntegerOverflow=on  OutDataTypeStr=Inherit: Same as first input
  force above slack length : Product  Inputs=**
  greater than slack length? : simulink/Logic and Bit Operations/Compare To Zero  relop=>  OutDataTypeStr=boolean  ZeroCross=off
  reference strain [lslack] : Constant  Value=mParams.muscles.eref
  relative strain : Product  Inputs=*/
  fse [Fmax] : Outport  VectorParamsAs1DForOutWhenUnconnected=off
  wires:
  force above slack length/1 -> fse [Fmax]/1
  greater than slack length?/1 -> force above slack length/1
  Sum4/1 -> relative strain/1, greater than slack length?/1
  reference strain [lslack]/1 -> relative strain/2
  relative strain/1 -> Math Function/1
  lse [lslack]/1 -> Sum4/1
  Math Function/1 -> force above slack length/2
  Constant1/1 -> Sum4/2
